simulink model "DconstPQ_snt"  (R2025b)
settings: Solver=ode45  StartTime=0.0  StopTime=10.0  RelTol=1e-3  EnableMultiTasking=on
undefined symbols (not defined in the file or in its folder): DiscIntNeverNeededParam, Ts
libraries: fl_lib x14, nesl_utility x14, mcbeeMathTransformLib x12, eeTransforms x12
(part 1 of 2)
settings Model: Creator=gdudgeon  LastModifiedBy=gdudgeon
settings SolverCC: AlgebraicLoopSolver=TrustRegion
settings DataIOCC: LimitDataPoints=on  SaveFormat=Array  ReturnWorkspaceOutputs=off
settings OptimizationCC: ExpressionDepthLimit=2147483647.0  LifeSpan=inf
settings DebuggingCC: UnderspecifiedInitializationDetection=Classic  MergeDetectMultiDrivingBlocksExec=none  SolverPrmCheckMsg=warning  UnconnectedInputMsg=warning  UnconnectedOutputMsg=warning  UnconnectedLineMsg=warning  StateNameClashWarn=warning  SFUnexpectedBacktrackingDiag=warning  SFNoUnconditionalDefaultTransitionDiag=warning  SFExecutionAtInitializationDiag=none  ArithmeticOperatorsInVariantConditions=warning
settings HardwareCC: ProdBitPerPointer=32.0  ProdBitPerSizeT=32.0  ProdBitPerPtrDiffT=32.0  ProdLargestAtomicFloat=None  ProdIntDivRoundTo=Undefined  ProdEndianess=Unspecified  ProdWordSize=32.0  ProdHWDeviceType=32-bit Generic
settings ModelReferenceCC: EnableRefExpFcnMdlSchedulingChecks=on  PropagateSignalLabelsOutOfModel=off
settings SFSimCC: SimUseLocalCustomCode=off  CustomCodeUndefinedFunction=UseInterfaceOnly
settings RTWCC: RTWUseLocalCustomCode=off  GPUComputeCapability=3.5
settings CodeAppCC: StateflowObjectComments=on
settings GRTTargetCC: TargetLangStandard=C89/C90 (ANSI)
settings ConfigComp: CovMetricSettings=dw  CovSaveCumulativeToWorkspaceVar=on  CovSaveSingleToWorkspaceVar=on  CovExternalEMLEnable=off  CovSFcnEnable=off
settings SimscapeCC: SimscapeNormalizeSystem=off

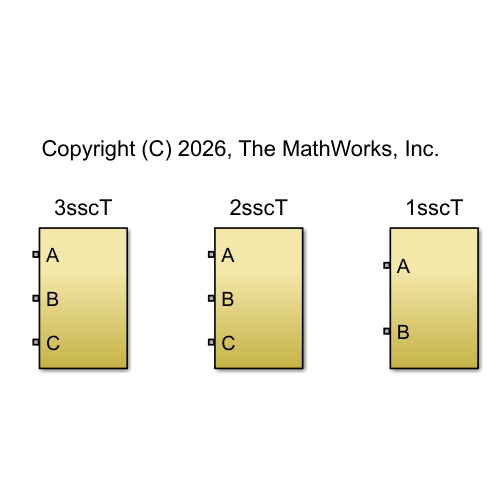
[thumbnail: Simulink's stored preview of the top-level diagram]
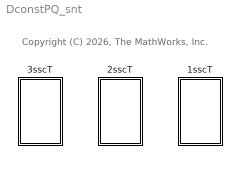
== system DconstPQ_snt ==
  note: Copyright (C) 2026, The MathWorks, Inc.
  1sscT : Subsystem
  2sscT : Subsystem
  3sscT : Subsystem

== system DconstPQ_snt/1sscT ==
  PQ1 : From
  constPQ1 : Subsystem
  A : PMIOPort  Side=Left
  B : PMIOPort  Port=2  Side=Left
  wires:
  PQ1/1 -> constPQ1/1(PQ)
  connections:
  constPQ1/LConn1 -- B/RConn1
  constPQ1/RConn1 -- A/RConn1

== system DconstPQ_snt/2sscT ==
  PQ1 : From
  PQ2 : From
  constPQ : Subsystem  Commented=on
  constPQ1 : Subsystem
  constPQ2 : Subsystem
  A : PMIOPort  Side=Left
  B : PMIOPort  Port=2  Side=Left
  C : PMIOPort  Port=3  Side=Left
  wires:
  PQ2/1 -> constPQ2/1(PQ)
  PQ1/1 -> constPQ1/1(PQ)
  connections:
  constPQ1/RConn1 -- A/RConn1
  B/RConn1 -- constPQ2/RConn1 -- constPQ1/LConn1
  constPQ2/LConn1 -- C/RConn1

== system DconstPQ_snt/3sscT ==
  PQ1 : From
  PQ2 : From
  PQ3 : From
  constPQ1 : Subsystem
  constPQ2 : Subsystem
  constPQ3 : Subsystem
  A : PMIOPort  Side=Left
  B : PMIOPort  Port=2  Side=Left
  C : PMIOPort  Port=3  Side=Left
  wires:
  PQ3/1 -> constPQ3/1(PQ)
  PQ2/1 -> constPQ2/1(PQ)
  PQ1/1 -> constPQ1/1(PQ)
  connections:
  C/RConn1 -- constPQ3/RConn1 -- constPQ2/LConn1
  B/RConn1 -- constPQ2/RConn1 -- constPQ1/LConn1
  A/RConn1 -- constPQ3/LConn1 -- constPQ1/RConn1

== system DconstPQ_snt/1sscT/constPQ1 ==
  PQ : Inport
  Controlled Current Source : fl_lib/Electrical/Electrical Sources/Controlled Current Source
  Demux : Demux  Outputs=2
  PS-Simulink Converter : nesl_utility/PS-Simulink Converter  PhysicalDomain=network_engine_domain  SubClassName=ps_output  LeftPortType=input  RightPortType=output  PseudoPeriodic=off  Frequencies=[]  VectorFormat=inherit  Unit=inherit  AffineConversion=off
  Simulink-PS Converter : nesl_utility/Simulink-PS Converter  PhysicalDomain=network_engine_domain  SubClassName=ps_input  LeftPortType=input  RightPortType=output  PseudoPeriodic=off  Frequencies=[]  NoiseDistribution=none  NoiseParameters=[]  Unit=1  AffineConversion=off  FilteringAndDerivatives=zero  SimscapeFilterOrder=1  InputFilterTimeConstant=0.001  UdotUserProvided=0
  Voltage Sensor : fl_lib/Electrical/Electrical Sensors/Voltage Sensor
  single-phase PQ : Subsystem
      settings: PortSchema="{\"entries\":[{\"content\":{\"sides\":[{\"content\":{\"connectorIds\":[\"In1\",\"In2\"]},\"type\":\"ConnectorPlacement.EquallySpacedRectSide\",\"uuid\":\"dcb77ad6-d65a-4afe-9b75-44cea2e03bc8\"},{\"content\":{\"connectorIds\":[\"Out1\"],\"side\":\"RIGHT\"},\"type\":\"ConnectorPlacement.EquallySpacedRectSide\",\"uuid\":\"20550ec8-912f-4e6b-8efc-55d7f6680ac4\"},{\"content\":{\"side\":\"TOP\"},\"type\":\"ConnectorPlacement.EquallySpacedRectSide\",\"uuid\":\"6ad8cbf4-1495-4620-97d9-4b8af34d00d1\"},{\"content\":{\"connectorIds\":[\"In3\"],\"side\":\"BOTTOM\"},\"type\":\"ConnectorPlacement.EquallySpacedRectSide\",\"uuid\":\"0b9a8788-8400-4a69-9d07-dd0028530e33\"}]},\"type\":\"ConnectorPlacement.EquallySpacedConnector\",\"uuid\":\"b57ec49b-aa32-43b3-a026-14ed90072d63\"}],\"packageUris\":[\"http://schema.mathworks.com/mf0/Connector/R2020b\"],\"version\":\"1.0\"}"
  + : PMIOPort  Side=Right
  - : PMIOPort  Port=2  Side=Left
  wires:
  PS-Simulink Converter/1 -> single-phase PQ/3(meas)
  single-phase PQ/1(I_1ph) -> Simulink-PS Converter/1
  Demux/1 -> single-phase PQ/1(P)
  Demux/2 -> single-phase PQ/2(Q)
  PQ/1 -> Demux/1
  connections:
  Controlled Current Source/RConn2 -- -/RConn1 -- Voltage Sensor/RConn2
  Voltage Sensor/LConn1 -- +/RConn1 -- Controlled Current Source/LConn1
  PS-Simulink Converter/LConn1 -- Voltage Sensor/RConn1
  Simulink-PS Converter/RConn1 -- Controlled Current Source/RConn1

== system DconstPQ_snt/2sscT/constPQ ==
  PQ : Inport
  Controlled Current Source : fl_lib/Electrical/Electrical Sources/Controlled Current Source
  Demux : Demux  Outputs=2
  PS-Simulink Converter : nesl_utility/PS-Simulink Converter  PhysicalDomain=network_engine_domain  SubClassName=ps_output  LeftPortType=input  RightPortType=output  PseudoPeriodic=off  Frequencies=[]  VectorFormat=inherit  Unit=inherit  AffineConversion=off
  Simulink-PS Converter : nesl_utility/Simulink-PS Converter  PhysicalDomain=network_engine_domain  SubClassName=ps_input  LeftPortType=input  RightPortType=output  PseudoPeriodic=off  Frequencies=[]  NoiseDistribution=none  NoiseParameters=[]  Unit=1  AffineConversion=off  FilteringAndDerivatives=zero  SimscapeFilterOrder=1  InputFilterTimeConstant=0.001  UdotUserProvided=0
  Voltage Sensor : fl_lib/Electrical/Electrical Sensors/Voltage Sensor
  single-phase PQ : Subsystem
      settings: PortSchema="{\"entries\":[{\"content\":{\"sides\":[{\"content\":{\"connectorIds\":[\"In1\",\"In2\"]},\"type\":\"ConnectorPlacement.EquallySpacedRectSide\",\"uuid\":\"dcb77ad6-d65a-4afe-9b75-44cea2e03bc8\"},{\"content\":{\"connectorIds\":[\"Out1\"],\"side\":\"RIGHT\"},\"type\":\"ConnectorPlacement.EquallySpacedRectSide\",\"uuid\":\"20550ec8-912f-4e6b-8efc-55d7f6680ac4\"},{\"content\":{\"side\":\"TOP\"},\"type\":\"ConnectorPlacement.EquallySpacedRectSide\",\"uuid\":\"6ad8cbf4-1495-4620-97d9-4b8af34d00d1\"},{\"content\":{\"connectorIds\":[\"In3\"],\"side\":\"BOTTOM\"},\"type\":\"ConnectorPlacement.EquallySpacedRectSide\",\"uuid\":\"0b9a8788-8400-4a69-9d07-dd0028530e33\"}]},\"type\":\"ConnectorPlacement.EquallySpacedConnector\",\"uuid\":\"b57ec49b-aa32-43b3-a026-14ed90072d63\"}],\"packageUris\":[\"http://schema.mathworks.com/mf0/Connector/R2020b\"],\"version\":\"1.0\"}"
  + : PMIOPort  Side=Right
  - : PMIOPort  Port=2  Side=Left
  wires:
  PS-Simulink Converter/1 -> single-phase PQ/3(meas)
  single-phase PQ/1(I_1ph) -> Simulink-PS Converter/1
  Demux/1 -> single-phase PQ/1(P)
  Demux/2 -> single-phase PQ/2(Q)
  PQ/1 -> Demux/1
  connections:
  Controlled Current Source/RConn2 -- -/RConn1 -- Voltage Sensor/RConn2
  Voltage Sensor/LConn1 -- +/RConn1 -- Controlled Current Source/LConn1
  PS-Simulink Converter/LConn1 -- Voltage Sensor/RConn1
  Simulink-PS Converter/RConn1 -- Controlled Current Source/RConn1

== system DconstPQ_snt/2sscT/constPQ1 ==
  PQ : Inport
  Controlled Current Source : fl_lib/Electrical/Electrical Sources/Controlled Current Source
  Demux : Demux  Outputs=2
  PS-Simulink Converter : nesl_utility/PS-Simulink Converter  PhysicalDomain=network_engine_domain  SubClassName=ps_output  LeftPortType=input  RightPortType=output  PseudoPeriodic=off  Frequencies=[]  VectorFormat=inherit  Unit=inherit  AffineConversion=off
  Simulink-PS Converter : nesl_utility/Simulink-PS Converter  PhysicalDomain=network_engine_domain  SubClassName=ps_input  LeftPortType=input  RightPortType=output  PseudoPeriodic=off  Frequencies=[]  NoiseDistribution=none  NoiseParameters=[]  Unit=1  AffineConversion=off  FilteringAndDerivatives=zero  SimscapeFilterOrder=1  InputFilterTimeConstant=0.001  UdotUserProvided=0
  Voltage Sensor : fl_lib/Electrical/Electrical Sensors/Voltage Sensor
  single-phase PQ : Subsystem
      settings: PortSchema="{\"entries\":[{\"content\":{\"sides\":[{\"content\":{\"connectorIds\":[\"In1\",\"In2\"]},\"type\":\"ConnectorPlacement.EquallySpacedRectSide\",\"uuid\":\"dcb77ad6-d65a-4afe-9b75-44cea2e03bc8\"},{\"content\":{\"connectorIds\":[\"Out1\"],\"side\":\"RIGHT\"},\"type\":\"ConnectorPlacement.EquallySpacedRectSide\",\"uuid\":\"20550ec8-912f-4e6b-8efc-55d7f6680ac4\"},{\"content\":{\"side\":\"TOP\"},\"type\":\"ConnectorPlacement.EquallySpacedRectSide\",\"uuid\":\"6ad8cbf4-1495-4620-97d9-4b8af34d00d1\"},{\"content\":{\"connectorIds\":[\"In3\"],\"side\":\"BOTTOM\"},\"type\":\"ConnectorPlacement.EquallySpacedRectSide\",\"uuid\":\"0b9a8788-8400-4a69-9d07-dd0028530e33\"}]},\"type\":\"ConnectorPlacement.EquallySpacedConnector\",\"uuid\":\"b57ec49b-aa32-43b3-a026-14ed90072d63\"}],\"packageUris\":[\"http://schema.mathworks.com/mf0/Connector/R2020b\"],\"version\":\"1.0\"}"
  + : PMIOPort  Side=Right
  - : PMIOPort  Port=2  Side=Left
  wires:
  PS-Simulink Converter/1 -> single-phase PQ/3(meas)
  single-phase PQ/1(I_1ph) -> Simulink-PS Converter/1
  Demux/1 -> single-phase PQ/1(P)
  Demux/2 -> single-phase PQ/2(Q)
  PQ/1 -> Demux/1
  connections:
  Controlled Current Source/RConn2 -- -/RConn1 -- Voltage Sensor/RConn2
  Voltage Sensor/LConn1 -- +/RConn1 -- Controlled Current Source/LConn1
  PS-Simulink Converter/LConn1 -- Voltage Sensor/RConn1
  Simulink-PS Converter/RConn1 -- Controlled Current Source/RConn1

== system DconstPQ_snt/2sscT/constPQ2 ==
  PQ : Inport
  Controlled Current Source : fl_lib/Electrical/Electrical Sources/Controlled Current Source
  Demux : Demux  Outputs=2
  PS-Simulink Converter : nesl_utility/PS-Simulink Converter  PhysicalDomain=network_engine_domain  SubClassName=ps_output  LeftPortType=input  RightPortType=output  PseudoPeriodic=off  Frequencies=[]  VectorFormat=inherit  Unit=inherit  AffineConversion=off
  Simulink-PS Converter : nesl_utility/Simulink-PS Converter  PhysicalDomain=network_engine_domain  SubClassName=ps_input  LeftPortType=input  RightPortType=output  PseudoPeriodic=off  Frequencies=[]  NoiseDistribution=none  NoiseParameters=[]  Unit=1  AffineConversion=off  FilteringAndDerivatives=zero  SimscapeFilterOrder=1  InputFilterTimeConstant=0.001  UdotUserProvided=0
  Voltage Sensor : fl_lib/Electrical/Electrical Sensors/Voltage Sensor
  single-phase PQ : Subsystem
      settings: PortSchema="{\"entries\":[{\"content\":{\"sides\":[{\"content\":{\"connectorIds\":[\"In1\",\"In2\"]},\"type\":\"ConnectorPlacement.EquallySpacedRectSide\",\"uuid\":\"dcb77ad6-d65a-4afe-9b75-44cea2e03bc8\"},{\"content\":{\"connectorIds\":[\"Out1\"],\"side\":\"RIGHT\"},\"type\":\"ConnectorPlacement.EquallySpacedRectSide\",\"uuid\":\"20550ec8-912f-4e6b-8efc-55d7f6680ac4\"},{\"content\":{\"side\":\"TOP\"},\"type\":\"ConnectorPlacement.EquallySpacedRectSide\",\"uuid\":\"6ad8cbf4-1495-4620-97d9-4b8af34d00d1\"},{\"content\":{\"connectorIds\":[\"In3\"],\"side\":\"BOTTOM\"},\"type\":\"ConnectorPlacement.EquallySpacedRectSide\",\"uuid\":\"0b9a8788-8400-4a69-9d07-dd0028530e33\"}]},\"type\":\"ConnectorPlacement.EquallySpacedConnector\",\"uuid\":\"b57ec49b-aa32-43b3-a026-14ed90072d63\"}],\"packageUris\":[\"http://schema.mathworks.com/mf0/Connector/R2020b\"],\"version\":\"1.0\"}"
  + : PMIOPort  Side=Right
  - : PMIOPort  Port=2  Side=Left
  wires:
  PQ/1 -> Demux/1
  Demux/2 -> single-phase PQ/2(Q)
  Demux/1 -> single-phase PQ/1(P)
  single-phase PQ/1(I_1ph) -> Simulink-PS Converter/1
  PS-Simulink Converter/1 -> single-phase PQ/3(meas)
  connections:
  Simulink-PS Converter/RConn1 -- Controlled Current Source/RConn1
  PS-Simulink Converter/LConn1 -- Voltage Sensor/RConn1
  Controlled Current Source/LConn1 -- +/RConn1 -- Voltage Sensor/LConn1
  Voltage Sensor/RConn2 -- -/RConn1 -- Controlled Current Source/RConn2

== system DconstPQ_snt/3sscT/constPQ1 ==
  PQ : Inport
  Controlled Current Source : fl_lib/Electrical/Electrical Sources/Controlled Current Source
  Demux : Demux  Outputs=2
  PS-Simulink Converter : nesl_utility/PS-Simulink Converter  PhysicalDomain=network_engine_domain  SubClassName=ps_output  LeftPortType=input  RightPortType=output  PseudoPeriodic=off  Frequencies=[]  VectorFormat=inherit  Unit=inherit  AffineConversion=off
  Simulink-PS Converter : nesl_utility/Simulink-PS Converter  PhysicalDomain=network_engine_domain  SubClassName=ps_input  LeftPortType=input  RightPortType=output  PseudoPeriodic=off  Frequencies=[]  NoiseDistribution=none  NoiseParameters=[]  Unit=1  AffineConversion=off  FilteringAndDerivatives=zero  SimscapeFilterOrder=1  InputFilterTimeConstant=0.001  UdotUserProvided=0
  Voltage Sensor : fl_lib/Electrical/Electrical Sensors/Voltage Sensor
  single-phase PQ : Subsystem
      settings: PortSchema="{\"entries\":[{\"content\":{\"sides\":[{\"content\":{\"connectorIds\":[\"In1\",\"In2\"]},\"type\":\"ConnectorPlacement.EquallySpacedRectSide\",\"uuid\":\"dcb77ad6-d65a-4afe-9b75-44cea2e03bc8\"},{\"content\":{\"connectorIds\":[\"Out1\"],\"side\":\"RIGHT\"},\"type\":\"ConnectorPlacement.EquallySpacedRectSide\",\"uuid\":\"20550ec8-912f-4e6b-8efc-55d7f6680ac4\"},{\"content\":{\"side\":\"TOP\"},\"type\":\"ConnectorPlacement.EquallySpacedRectSide\",\"uuid\":\"6ad8cbf4-1495-4620-97d9-4b8af34d00d1\"},{\"content\":{\"connectorIds\":[\"In3\"],\"side\":\"BOTTOM\"},\"type\":\"ConnectorPlacement.EquallySpacedRectSide\",\"uuid\":\"0b9a8788-8400-4a69-9d07-dd0028530e33\"}]},\"type\":\"ConnectorPlacement.EquallySpacedConnector\",\"uuid\":\"b57ec49b-aa32-43b3-a026-14ed90072d63\"}],\"packageUris\":[\"http://schema.mathworks.com/mf0/Connector/R2020b\"],\"version\":\"1.0\"}"
  + : PMIOPort  Side=Right
  - : PMIOPort  Port=2  Side=Left
  wires:
  PS-Simulink Converter/1 -> single-phase PQ/3(meas)
  single-phase PQ/1(I_1ph) -> Simulink-PS Converter/1
  Demux/1 -> single-phase PQ/1(P)
  Demux/2 -> single-phase PQ/2(Q)
  PQ/1 -> Demux/1
  connections:
  Controlled Current Source/RConn2 -- -/RConn1 -- Voltage Sensor/RConn2
  Voltage Sensor/LConn1 -- +/RConn1 -- Controlled Current Source/LConn1
  PS-Simulink Converter/LConn1 -- Voltage Sensor/RConn1
  Simulink-PS Converter/RConn1 -- Controlled Current Source/RConn1

== system DconstPQ_snt/3sscT/constPQ2 ==
  PQ : Inport
  Controlled Current Source : fl_lib/Electrical/Electrical Sources/Controlled Current Source
  Demux : Demux  Outputs=2
  PS-Simulink Converter : nesl_utility/PS-Simulink Converter  PhysicalDomain=network_engine_domain  SubClassName=ps_output  LeftPortType=input  RightPortType=output  PseudoPeriodic=off  Frequencies=[]  VectorFormat=inherit  Unit=inherit  AffineConversion=off
  Simulink-PS Converter : nesl_utility/Simulink-PS Converter  PhysicalDomain=network_engine_domain  SubClassName=ps_input  LeftPortType=input  RightPortType=output  PseudoPeriodic=off  Frequencies=[]  NoiseDistribution=none  NoiseParameters=[]  Unit=1  AffineConversion=off  FilteringAndDerivatives=zero  SimscapeFilterOrder=1  InputFilterTimeConstant=0.001  UdotUserProvided=0
  Voltage Sensor : fl_lib/Electrical/Electrical Sensors/Voltage Sensor
  single-phase PQ : Subsystem
      settings: PortSchema="{\"entries\":[{\"content\":{\"sides\":[{\"content\":{\"connectorIds\":[\"In1\",\"In2\"]},\"type\":\"ConnectorPlacement.EquallySpacedRectSide\",\"uuid\":\"dcb77ad6-d65a-4afe-9b75-44cea2e03bc8\"},{\"content\":{\"connectorIds\":[\"Out1\"],\"side\":\"RIGHT\"},\"type\":\"ConnectorPlacement.EquallySpacedRectSide\",\"uuid\":\"20550ec8-912f-4e6b-8efc-55d7f6680ac4\"},{\"content\":{\"side\":\"TOP\"},\"type\":\"ConnectorPlacement.EquallySpacedRectSide\",\"uuid\":\"6ad8cbf4-1495-4620-97d9-4b8af34d00d1\"},{\"content\":{\"connectorIds\":[\"In3\"],\"side\":\"BOTTOM\"},\"type\":\"ConnectorPlacement.EquallySpacedRectSide\",\"uuid\":\"0b9a8788-8400-4a69-9d07-dd0028530e33\"}]},\"type\":\"ConnectorPlacement.EquallySpacedConnector\",\"uuid\":\"b57ec49b-aa32-43b3-a026-14ed90072d63\"}],\"packageUris\":[\"http://schema.mathworks.com/mf0/Connector/R2020b\"],\"version\":\"1.0\"}"
  + : PMIOPort  Side=Right
  - : PMIOPort  Port=2  Side=Left
  wires:
  PQ/1 -> Demux/1
  Demux/2 -> single-phase PQ/2(Q)
  Demux/1 -> single-phase PQ/1(P)
  single-phase PQ/1(I_1ph) -> Simulink-PS Converter/1
  PS-Simulink Converter/1 -> single-phase PQ/3(meas)
  connections:
  Simulink-PS Converter/RConn1 -- Controlled Current Source/RConn1
  PS-Simulink Converter/LConn1 -- Voltage Sensor/RConn1
  Controlled Current Source/LConn1 -- +/RConn1 -- Voltage Sensor/LConn1
  Voltage Sensor/RConn2 -- -/RConn1 -- Controlled Current Source/RConn2

== system DconstPQ_snt/3sscT/constPQ3 ==
  PQ : Inport
  Controlled Current Source : fl_lib/Electrical/Electrical Sources/Controlled Current Source
  Demux : Demux  Outputs=2
  PS-Simulink Converter : nesl_utility/PS-Simulink Converter  PhysicalDomain=network_engine_domain  SubClassName=ps_output  LeftPortType=input  RightPortType=output  PseudoPeriodic=off  Frequencies=[]  VectorFormat=inherit  Unit=inherit  AffineConversion=off
  Simulink-PS Converter : nesl_utility/Simulink-PS Converter  PhysicalDomain=network_engine_domain  SubClassName=ps_input  LeftPortType=input  RightPortType=output  PseudoPeriodic=off  Frequencies=[]  NoiseDistribution=none  NoiseParameters=[]  Unit=1  AffineConversion=off  FilteringAndDerivatives=zero  SimscapeFilterOrder=1  InputFilterTimeConstant=0.001  UdotUserProvided=0
  Voltage Sensor : fl_lib/Electrical/Electrical Sensors/Voltage Sensor
  single-phase PQ : Subsystem
      settings: PortSchema="{\"entries\":[{\"content\":{\"sides\":[{\"content\":{\"connectorIds\":[\"In1\",\"In2\"]},\"type\":\"ConnectorPlacement.EquallySpacedRectSide\",\"uuid\":\"dcb77ad6-d65a-4afe-9b75-44cea2e03bc8\"},{\"content\":{\"connectorIds\":[\"Out1\"],\"side\":\"RIGHT\"},\"type\":\"ConnectorPlacement.EquallySpacedRectSide\",\"uuid\":\"20550ec8-912f-4e6b-8efc-55d7f6680ac4\"},{\"content\":{\"side\":\"TOP\"},\"type\":\"ConnectorPlacement.EquallySpacedRectSide\",\"uuid\":\"6ad8cbf4-1495-4620-97d9-4b8af34d00d1\"},{\"content\":{\"connectorIds\":[\"In3\"],\"side\":\"BOTTOM\"},\"type\":\"ConnectorPlacement.EquallySpacedRectSide\",\"uuid\":\"0b9a8788-8400-4a69-9d07-dd0028530e33\"}]},\"type\":\"ConnectorPlacement.EquallySpacedConnector\",\"uuid\":\"b57ec49b-aa32-43b3-a026-14ed90072d63\"}],\"packageUris\":[\"http://schema.mathworks.com/mf0/Connector/R2020b\"],\"version\":\"1.0\"}"
  + : PMIOPort  Side=Right
  - : PMIOPort  Port=2  Side=Left
  wires:
  PS-Simulink Converter/1 -> single-phase PQ/3(meas)
  single-phase PQ/1(I_1ph) -> Simulink-PS Converter/1
  Demux/1 -> single-phase PQ/1(P)
  Demux/2 -> single-phase PQ/2(Q)
  PQ/1 -> Demux/1
  connections:
  Controlled Current Source/RConn2 -- -/RConn1 -- Voltage Sensor/RConn2
  Voltage Sensor/LConn1 -- +/RConn1 -- Controlled Current Source/LConn1
  PS-Simulink Converter/LConn1 -- Voltage Sensor/RConn1
  Simulink-PS Converter/RConn1 -- Controlled Current Source/RConn1

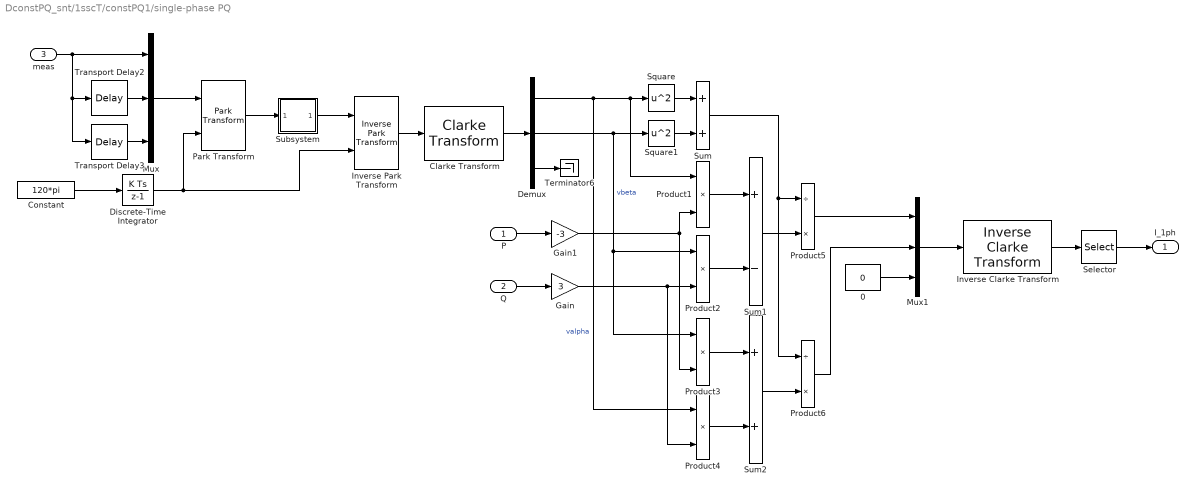
== system DconstPQ_snt/1sscT/constPQ1/single-phase PQ ==
  P : Inport
  Q : Inport  Port=2
  meas : Inport  Port=3
  "0 " : Constant  Value=0  VectorParams1D=off  SampleTime=Ts
  Clarke Transform : mcbeeMathTransformLib/Clarke Transform  PowerInvariant=on  UseWithEmbedded=off  PhaseInput=Two inputs
      settings: LibrarySourceBlock=|
      | ee_sl_lib/Mathematical
      | Transforms/Clarke Transform
  Constant : Constant  Value=120*pi  VectorParams1D=off  SampleTime=Ts
  Demux : Demux  Outputs=3
  Discrete-Time Integrator : DiscreteIntegrator  SampleTime=Ts  ICPrevOutput=DiscIntNeverNeededParam  ICPrevScaledInput=DiscIntNeverNeededParam
  Gain : Gain  Gain=3
  Gain1 : Gain  Gain=-3
  Inverse Clarke Transform : mcbeeMathTransformLib/Inverse Clarke Transform  PowerInvariant=on  UseWithEmbedded=off  PhaseInput=Two inputs
      settings: LibrarySourceBlock=|
      | ee_sl_lib/Mathematical
      | Transforms/Inverse
      | Clarke Transform
  Inverse Park Transform : eeTransforms/Inverse Park Transform  AxisAlignment=Q-axis  PowerInvariant=off
      settings: LibrarySourceBlock=|
      | ee_sl_lib/Mathematical
      | Transforms/Inverse
      | Park Transform
  Mux : Mux  Inputs=3
  Mux1 : Mux  Inputs=3
  Park Transform : eeTransforms/Park Transform  AxisAlignment=Q-axis  PowerInvariant=off
      settings: LibrarySourceBlock=|
      | ee_sl_lib/Mathematical
      | Transforms/Park Transform
  Product{1..4} (4 alike) : Product
  Product5 : Product  Inputs=/*
  Product6 : Product  Inputs=/*
  Selector : Selector  InputPortWidth=3  IndexOptions=Index vector (dialog)  Indices=1  OutputSizes=1
  Square : Math  Operator=square
  Square1 : Math  Operator=square
  Subsystem : Subsystem
  Sum : Sum
  Sum1 : Sum  Inputs=+-
  Sum2 : Sum
  Terminator6 : Terminator
  Transport Delay2 : TransportDelay  DelayTime=1/180
  Transport Delay3 : TransportDelay  DelayTime=2/180
  I_1ph : Outport
  wires:
  Sum2/1 -> Product6/2
  Sum/1 -> Product5/1, Product6/1
  P/1 -> Gain1/1
  Square1/1 -> Sum/2
  Product3/1 -> Sum2/1
  Demux/2 -> Product3/1, Product2/1, Square1/1  "vbeta"
  Q/1 -> Gain/1
  "0 "/1 -> Mux1/3
  Sum1/1 -> Product5/2
  Product2/1 -> Sum1/2
  Demux/1 -> Product4/1, Product1/1, Square/1  "valpha"
  Product6/1 -> Mux1/2
  Product4/1 -> Sum2/2
  Product1/1 -> Sum1/1
  Square/1 -> Sum/1
  Product5/1 -> Mux1/1
  Constant/1 -> Discrete-Time Integrator/1
  Discrete-Time Integrator/1 -> Park Transform/2, Inverse Park Transform/2
  Subsystem/1(Out1) -> Inverse Park Transform/1
  Transport Delay3/1 -> Mux/3
  meas/1 -> Transport Delay3/1, Transport Delay2/1, Mux/1
  Transport Delay2/1 -> Mux/2
  Gain/1 -> Product4/2, Product2/2
  Gain1/1 -> Product1/2, Product3/2
  Mux/1 -> Park Transform/1
  Selector/1 -> I_1ph/1
  Park Transform/1 -> Subsystem/1(In1)
  Inverse Park Transform/1 -> Clarke Transform/1
  Clarke Transform/1 -> Demux/1
  Demux/3 -> Terminator6/1
  Mux1/1 -> Inverse Clarke Transform/1
  Inverse Clarke Transform/1 -> Selector/1

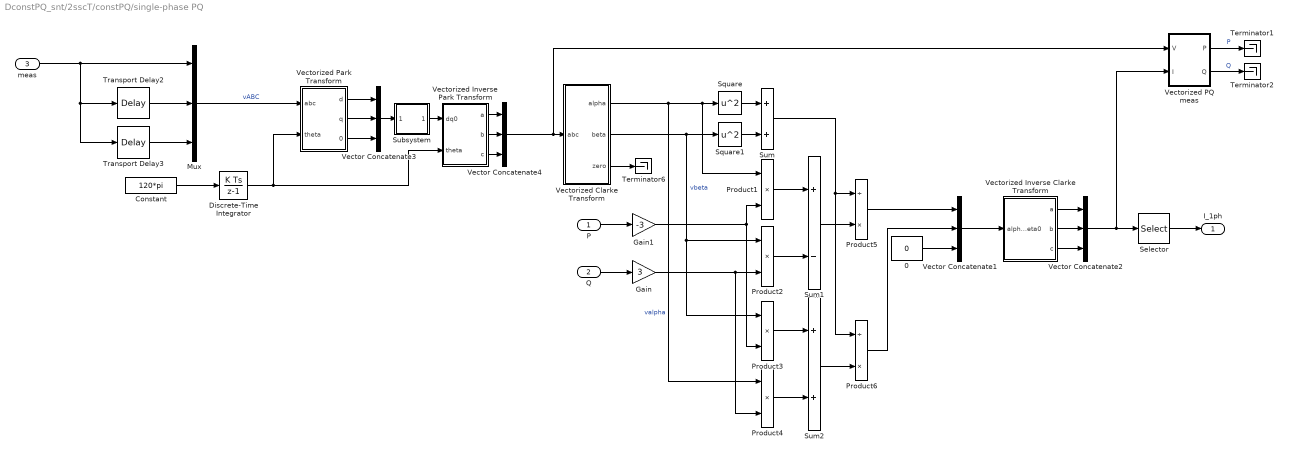
== system DconstPQ_snt/2sscT/constPQ/single-phase PQ ==
  P : Inport
  Q : Inport  Port=2
  meas : Inport  Port=3
  "0 " : Constant  Value=0  VectorParams1D=off  SampleTime=Ts
  Constant : Constant  Value=120*pi  VectorParams1D=off  SampleTime=Ts
  Discrete-Time Integrator : DiscreteIntegrator  SampleTime=Ts  ICPrevOutput=DiscIntNeverNeededParam  ICPrevScaledInput=DiscIntNeverNeededParam
  Gain : Gain  Gain=3
  Gain1 : Gain  Gain=-3
  Mux : Mux  Inputs=3
  Product{1..4} (4 alike) : Product
  Product5 : Product  Inputs=/*
  Product6 : Product  Inputs=/*
  Selector : Selector  InputPortWidth=3  IndexOptions=Index vector (dialog)  Indices=1  OutputSizes=1
  Square : Math  Operator=square
  Square1 : Math  Operator=square
  Subsystem : Subsystem
  Sum : Sum
  Sum1 : Sum  Inputs=+-
  Sum2 : Sum
  Terminator1 : Terminator
  Terminator2 : Terminator
  Terminator6 : Terminator
  Transport Delay2 : TransportDelay  DelayTime=1/180
  Transport Delay3 : TransportDelay  DelayTime=2/180
  Vector Concatenate{1..4} (4 alike) : Concatenate  NumInputs=3  Mode=Multidimensional array
  Vectorized Clarke Transform : Subsystem  mask{no_meas=1}
      mask prompts: no_meas "Number of measurements"
  Vectorized PQ meas : Subsystem  DialogController=POWERSYS.PowerSysDialog
  Vectorized Park Transform : Subsystem  mask{no_meas=1}
      mask prompts: no_meas "Number of measurements"
  Vectorized Inverse Clarke Transform : Subsystem  mask{no_meas=1}
      mask prompts: no_meas "Number of Measurements"
      mask Display:
      | port_label('input', 1, '\alpha\beta0', 'texmode', 'on')
      | port_label('output',1,'a')
      | port_label('output',2,'b')
      | port_label('output',3,'c')
  Vectorized Inverse Park Transform : Subsystem  mask{no_meas=1}
      mask prompts: no_meas "Number of Measurements"
  I_1ph : Outport
  wires:
  Sum2/1 -> Product6/2
  Sum/1 -> Product5/1, Product6/1
  P/1 -> Gain1/1
  Square1/1 -> Sum/2
  Product3/1 -> Sum2/1
  Vectorized Clarke Transform/2(beta) -> Product3/1, Product2/1, Square1/1  "vbeta"
  Q/1 -> Gain/1
  "0 "/1 -> Vector Concatenate1/3
  Sum1/1 -> Product5/2
  Vectorized Inverse Clarke Transform/1(a) -> Vector Concatenate2/1
  Vectorized Inverse Clarke Transform/2(b) -> Vector Concatenate2/2
  Vectorized Clarke Transform/3(zero) -> Terminator6/1
  Product2/1 -> Sum1/2
  Vectorized Clarke Transform/1(alpha) -> Product4/1, Product1/1, Square/1  "valpha"
  Product6/1 -> Vector Concatenate1/2
  Product4/1 -> Sum2/2
  Vectorized Inverse Clarke Transform/3(c) -> Vector Concatenate2/3
  Product1/1 -> Sum1/1
  Vector Concatenate1/1 -> Vectorized Inverse Clarke Transform/1(alphabeta0)
  Square/1 -> Sum/1
  Product5/1 -> Vector Concatenate1/1
  Vectorized PQ meas/1(P) -> Terminator1/1  "P"
  Vectorized PQ meas/2(Q) -> Terminator2/1  "Q"
  Vector Concatenate2/1 -> Selector/1, Vectorized PQ meas/2(I)
  Vectorized Park Transform/1(d) -> Vector Concatenate3/1
  Vectorized Park Transform/2(q) -> Vector Concatenate3/2
  Vectorized Park Transform/3(0) -> Vector Concatenate3/3
  Vectorized Inverse Park Transform/1(a) -> Vector Concatenate4/1
  Vectorized Inverse Park Transform/2(b) -> Vector Concatenate4/2
  Vectorized Inverse Park Transform/3(c) -> Vector Concatenate4/3
  Vector Concatenate4/1 -> Vectorized Clarke Transform/1(abc), Vectorized PQ meas/1(V)
  Constant/1 -> Discrete-Time Integrator/1
  Discrete-Time Integrator/1 -> Vectorized Inverse Park Transform/2(theta), Vectorized Park Transform/2(theta)
  Vector Concatenate3/1 -> Subsystem/1(In1)
  Subsystem/1(Out1) -> Vectorized Inverse Park Transform/1(dq0)
  Transport Delay3/1 -> Mux/3
  meas/1 -> Transport Delay3/1, Transport Delay2/1, Mux/1
  Transport Delay2/1 -> Mux/2
  Gain/1 -> Product4/2, Product2/2
  Gain1/1 -> Product1/2, Product3/2
  Mux/1 -> Vectorized Park Transform/1(abc)  "vABC"
  Selector/1 -> I_1ph/1

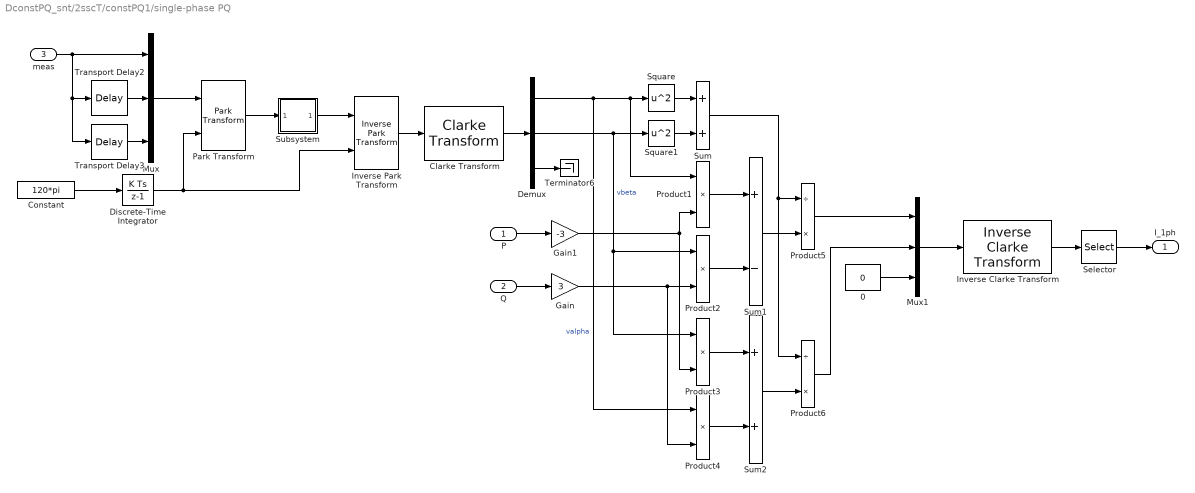
== system DconstPQ_snt/2sscT/constPQ1/single-phase PQ ==
  P : Inport
  Q : Inport  Port=2
  meas : Inport  Port=3
  "0 " : Constant  Value=0  VectorParams1D=off  SampleTime=Ts
  Clarke Transform : mcbeeMathTransformLib/Clarke Transform  PowerInvariant=on  UseWithEmbedded=off  PhaseInput=Two inputs
      settings: LibrarySourceBlock=|
      | ee_sl_lib/Mathematical
      | Transforms/Clarke Transform
  Constant : Constant  Value=120*pi  VectorParams1D=off  SampleTime=Ts
  Demux : Demux  Outputs=3
  Discrete-Time Integrator : DiscreteIntegrator  SampleTime=Ts  ICPrevOutput=DiscIntNeverNeededParam  ICPrevScaledInput=DiscIntNeverNeededParam
  Gain : Gain  Gain=3
  Gain1 : Gain  Gain=-3
  Inverse Clarke Transform : mcbeeMathTransformLib/Inverse Clarke Transform  PowerInvariant=on  UseWithEmbedded=off  PhaseInput=Two inputs
      settings: LibrarySourceBlock=|
      | ee_sl_lib/Mathematical
      | Transforms/Inverse
      | Clarke Transform
  Inverse Park Transform : eeTransforms/Inverse Park Transform  AxisAlignment=Q-axis  PowerInvariant=off
      settings: LibrarySourceBlock=|
      | ee_sl_lib/Mathematical
      | Transforms/Inverse
      | Park Transform
  Mux : Mux  Inputs=3
  Mux1 : Mux  Inputs=3
  Park Transform : eeTransforms/Park Transform  AxisAlignment=Q-axis  PowerInvariant=off
      settings: LibrarySourceBlock=|
      | ee_sl_lib/Mathematical
      | Transforms/Park Transform
  Product{1..4} (4 alike) : Product
  Product5 : Product  Inputs=/*
  Product6 : Product  Inputs=/*
  Selector : Selector  InputPortWidth=3  IndexOptions=Index vector (dialog)  Indices=1  OutputSizes=1
  Square : Math  Operator=square
  Square1 : Math  Operator=square
  Subsystem : Subsystem
  Sum : Sum
  Sum1 : Sum  Inputs=+-
  Sum2 : Sum
  Terminator6 : Terminator
  Transport Delay2 : TransportDelay  DelayTime=1/180
  Transport Delay3 : TransportDelay  DelayTime=2/180
  I_1ph : Outport
  wires:
  Sum2/1 -> Product6/2
  Sum/1 -> Product5/1, Product6/1
  P/1 -> Gain1/1
  Square1/1 -> Sum/2
  Product3/1 -> Sum2/1
  Demux/2 -> Product3/1, Product2/1, Square1/1  "vbeta"
  Q/1 -> Gain/1
  "0 "/1 -> Mux1/3
  Sum1/1 -> Product5/2
  Product2/1 -> Sum1/2
  Demux/1 -> Product4/1, Product1/1, Square/1  "valpha"
  Product6/1 -> Mux1/2
  Product4/1 -> Sum2/2
  Product1/1 -> Sum1/1
  Square/1 -> Sum/1
  Product5/1 -> Mux1/1
  Constant/1 -> Discrete-Time Integrator/1
  Discrete-Time Integrator/1 -> Park Transform/2, Inverse Park Transform/2
  Subsystem/1(Out1) -> Inverse Park Transform/1
  Transport Delay3/1 -> Mux/3
  meas/1 -> Transport Delay3/1, Transport Delay2/1, Mux/1
  Transport Delay2/1 -> Mux/2
  Gain/1 -> Product4/2, Product2/2
  Gain1/1 -> Product1/2, Product3/2
  Mux/1 -> Park Transform/1
  Selector/1 -> I_1ph/1
  Park Transform/1 -> Subsystem/1(In1)
  Inverse Park Transform/1 -> Clarke Transform/1
  Clarke Transform/1 -> Demux/1
  Demux/3 -> Terminator6/1
  Mux1/1 -> Inverse Clarke Transform/1
  Inverse Clarke Transform/1 -> Selector/1

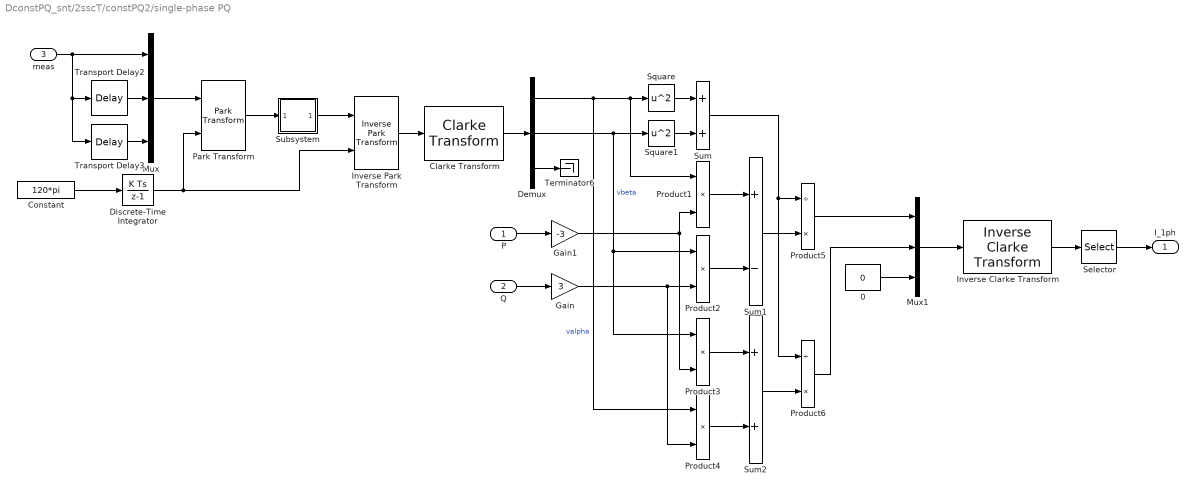
== system DconstPQ_snt/2sscT/constPQ2/single-phase PQ ==
  P : Inport
  Q : Inport  Port=2
  meas : Inport  Port=3
  "0 " : Constant  Value=0  VectorParams1D=off  SampleTime=Ts
  Clarke Transform : mcbeeMathTransformLib/Clarke Transform  PowerInvariant=on  UseWithEmbedded=off  PhaseInput=Two inputs
      settings: LibrarySourceBlock=|
      | ee_sl_lib/Mathematical
      | Transforms/Clarke Transform
  Constant : Constant  Value=120*pi  VectorParams1D=off  SampleTime=Ts
  Demux : Demux  Outputs=3
  Discrete-Time Integrator : DiscreteIntegrator  SampleTime=Ts  ICPrevOutput=DiscIntNeverNeededParam  ICPrevScaledInput=DiscIntNeverNeededParam
  Gain : Gain  Gain=3
  Gain1 : Gain  Gain=-3
  Inverse Clarke Transform : mcbeeMathTransformLib/Inverse Clarke Transform  PowerInvariant=on  UseWithEmbedded=off  PhaseInput=Two inputs
      settings: LibrarySourceBlock=|
      | ee_sl_lib/Mathematical
      | Transforms/Inverse
      | Clarke Transform
  Inverse Park Transform : eeTransforms/Inverse Park Transform  AxisAlignment=Q-axis  PowerInvariant=off
      settings: LibrarySourceBlock=|
      | ee_sl_lib/Mathematical
      | Transforms/Inverse
      | Park Transform
  Mux : Mux  Inputs=3
  Mux1 : Mux  Inputs=3
  Park Transform : eeTransforms/Park Transform  AxisAlignment=Q-axis  PowerInvariant=off
      settings: LibrarySourceBlock=|
      | ee_sl_lib/Mathematical
      | Transforms/Park Transform
  Product{1..4} (4 alike) : Product
  Product5 : Product  Inputs=/*
  Product6 : Product  Inputs=/*
  Selector : Selector  InputPortWidth=3  IndexOptions=Index vector (dialog)  Indices=1  OutputSizes=1
  Square : Math  Operator=square
  Square1 : Math  Operator=square
  Subsystem : Subsystem
  Sum : Sum
  Sum1 : Sum  Inputs=+-
  Sum2 : Sum
  Terminator6 : Terminator
  Transport Delay2 : TransportDelay  DelayTime=1/180
  Transport Delay3 : TransportDelay  DelayTime=2/180
  I_1ph : Outport
  wires:
  Inverse Clarke Transform/1 -> Selector/1
  Mux1/1 -> Inverse Clarke Transform/1
  Demux/3 -> Terminator6/1
  Clarke Transform/1 -> Demux/1
  Inverse Park Transform/1 -> Clarke Transform/1
  Park Transform/1 -> Subsystem/1(In1)
  Selector/1 -> I_1ph/1
  Mux/1 -> Park Transform/1
  Gain1/1 -> Product3/2, Product1/2
  Gain/1 -> Product2/2, Product4/2
  Transport Delay2/1 -> Mux/2
  meas/1 -> Mux/1, Transport Delay2/1, Transport Delay3/1
  Transport Delay3/1 -> Mux/3
  Subsystem/1(Out1) -> Inverse Park Transform/1
  Discrete-Time Integrator/1 -> Inverse Park Transform/2, Park Transform/2
  Constant/1 -> Discrete-Time Integrator/1
  Product5/1 -> Mux1/1
  Square/1 -> Sum/1
  Product1/1 -> Sum1/1
  Product4/1 -> Sum2/2
  Product6/1 -> Mux1/2
  Demux/1 -> Square/1, Product1/1, Product4/1  "valpha"
  Product2/1 -> Sum1/2
  Sum1/1 -> Product5/2
  "0 "/1 -> Mux1/3
  Q/1 -> Gain/1
  Demux/2 -> Square1/1, Product2/1, Product3/1  "vbeta"
  Product3/1 -> Sum2/1
  Square1/1 -> Sum/2
  P/1 -> Gain1/1
  Sum/1 -> Product6/1, Product5/1
  Sum2/1 -> Product6/2

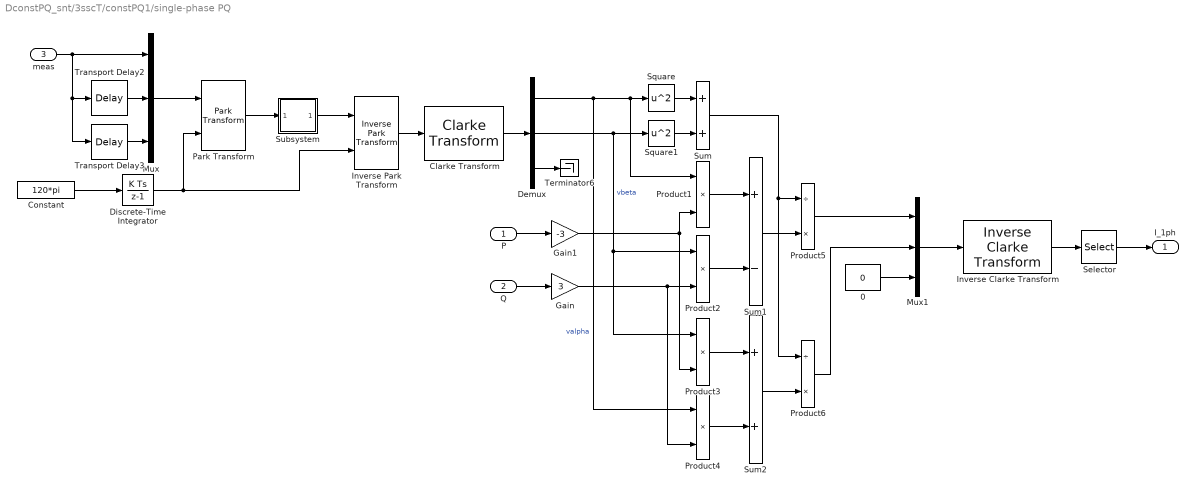
== system DconstPQ_snt/3sscT/constPQ1/single-phase PQ ==
  P : Inport
  Q : Inport  Port=2
  meas : Inport  Port=3
  "0 " : Constant  Value=0  VectorParams1D=off  SampleTime=Ts
  Clarke Transform : mcbeeMathTransformLib/Clarke Transform  PowerInvariant=on  UseWithEmbedded=off  PhaseInput=Two inputs
      settings: LibrarySourceBlock=|
      | ee_sl_lib/Mathematical
      | Transforms/Clarke Transform
  Constant : Constant  Value=120*pi  VectorParams1D=off  SampleTime=Ts
  Demux : Demux  Outputs=3
  Discrete-Time Integrator : DiscreteIntegrator  SampleTime=Ts  ICPrevOutput=DiscIntNeverNeededParam  ICPrevScaledInput=DiscIntNeverNeededParam
  Gain : Gain  Gain=3
  Gain1 : Gain  Gain=-3
  Inverse Clarke Transform : mcbeeMathTransformLib/Inverse Clarke Transform  PowerInvariant=on  UseWithEmbedded=off  PhaseInput=Two inputs
      settings: LibrarySourceBlock=|
      | ee_sl_lib/Mathematical
      | Transforms/Inverse
      | Clarke Transform
  Inverse Park Transform : eeTransforms/Inverse Park Transform  AxisAlignment=Q-axis  PowerInvariant=off
      settings: LibrarySourceBlock=|
      | ee_sl_lib/Mathematical
      | Transforms/Inverse
      | Park Transform
  Mux : Mux  Inputs=3
  Mux1 : Mux  Inputs=3
  Park Transform : eeTransforms/Park Transform  AxisAlignment=Q-axis  PowerInvariant=off
      settings: LibrarySourceBlock=|
      | ee_sl_lib/Mathematical
      | Transforms/Park Transform
  Product{1..4} (4 alike) : Product
  Product5 : Product  Inputs=/*
  Product6 : Product  Inputs=/*
  Selector : Selector  InputPortWidth=3  IndexOptions=Index vector (dialog)  Indices=1  OutputSizes=1
  Square : Math  Operator=square
  Square1 : Math  Operator=square
  Subsystem : Subsystem
  Sum : Sum
  Sum1 : Sum  Inputs=+-
  Sum2 : Sum
  Terminator6 : Terminator
  Transport Delay2 : TransportDelay  DelayTime=1/180
  Transport Delay3 : TransportDelay  DelayTime=2/180
  I_1ph : Outport
  wires:
  Sum2/1 -> Product6/2
  Sum/1 -> Product5/1, Product6/1
  P/1 -> Gain1/1
  Square1/1 -> Sum/2
  Product3/1 -> Sum2/1
  Demux/2 -> Product3/1, Product2/1, Square1/1  "vbeta"
  Q/1 -> Gain/1
  "0 "/1 -> Mux1/3
  Sum1/1 -> Product5/2
  Product2/1 -> Sum1/2
  Demux/1 -> Product4/1, Product1/1, Square/1  "valpha"
  Product6/1 -> Mux1/2
  Product4/1 -> Sum2/2
  Product1/1 -> Sum1/1
  Square/1 -> Sum/1
  Product5/1 -> Mux1/1
  Constant/1 -> Discrete-Time Integrator/1
  Discrete-Time Integrator/1 -> Park Transform/2, Inverse Park Transform/2
  Subsystem/1(Out1) -> Inverse Park Transform/1
  Transport Delay3/1 -> Mux/3
  meas/1 -> Transport Delay3/1, Transport Delay2/1, Mux/1
  Transport Delay2/1 -> Mux/2
  Gain/1 -> Product4/2, Product2/2
  Gain1/1 -> Product1/2, Product3/2
  Mux/1 -> Park Transform/1
  Selector/1 -> I_1ph/1
  Park Transform/1 -> Subsystem/1(In1)
  Inverse Park Transform/1 -> Clarke Transform/1
  Clarke Transform/1 -> Demux/1
  Demux/3 -> Terminator6/1
  Mux1/1 -> Inverse Clarke Transform/1
  Inverse Clarke Transform/1 -> Selector/1

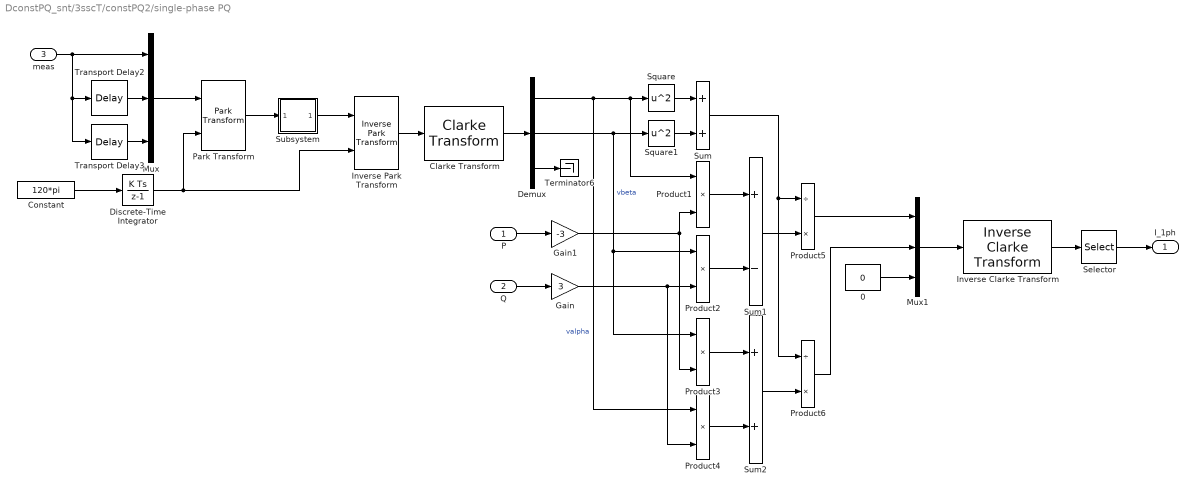
== system DconstPQ_snt/3sscT/constPQ2/single-phase PQ ==
  P : Inport
  Q : Inport  Port=2
  meas : Inport  Port=3
  "0 " : Constant  Value=0  VectorParams1D=off  SampleTime=Ts
  Clarke Transform : mcbeeMathTransformLib/Clarke Transform  PowerInvariant=on  UseWithEmbedded=off  PhaseInput=Two inputs
      settings: LibrarySourceBlock=|
      | ee_sl_lib/Mathematical
      | Transforms/Clarke Transform
  Constant : Constant  Value=120*pi  VectorParams1D=off  SampleTime=Ts
  Demux : Demux  Outputs=3
  Discrete-Time Integrator : DiscreteIntegrator  SampleTime=Ts  ICPrevOutput=DiscIntNeverNeededParam  ICPrevScaledInput=DiscIntNeverNeededParam
  Gain : Gain  Gain=3
  Gain1 : Gain  Gain=-3
  Inverse Clarke Transform : mcbeeMathTransformLib/Inverse Clarke Transform  PowerInvariant=on  UseWithEmbedded=off  PhaseInput=Two inputs
      settings: LibrarySourceBlock=|
      | ee_sl_lib/Mathematical
      | Transforms/Inverse
      | Clarke Transform
  Inverse Park Transform : eeTransforms/Inverse Park Transform  AxisAlignment=Q-axis  PowerInvariant=off
      settings: LibrarySourceBlock=|
      | ee_sl_lib/Mathematical
      | Transforms/Inverse
      | Park Transform
  Mux : Mux  Inputs=3
  Mux1 : Mux  Inputs=3
  Park Transform : eeTransforms/Park Transform  AxisAlignment=Q-axis  PowerInvariant=off
      settings: LibrarySourceBlock=|
      | ee_sl_lib/Mathematical
      | Transforms/Park Transform
  Product{1..4} (4 alike) : Product
  Product5 : Product  Inputs=/*
  Product6 : Product  Inputs=/*
  Selector : Selector  InputPortWidth=3  IndexOptions=Index vector (dialog)  Indices=1  OutputSizes=1
  Square : Math  Operator=square
  Square1 : Math  Operator=square
  Subsystem : Subsystem
  Sum : Sum
  Sum1 : Sum  Inputs=+-
  Sum2 : Sum
  Terminator6 : Terminator
  Transport Delay2 : TransportDelay  DelayTime=1/180
  Transport Delay3 : TransportDelay  DelayTime=2/180
  I_1ph : Outport
  wires:
  Inverse Clarke Transform/1 -> Selector/1
  Mux1/1 -> Inverse Clarke Transform/1
  Demux/3 -> Terminator6/1
  Clarke Transform/1 -> Demux/1
  Inverse Park Transform/1 -> Clarke Transform/1
  Park Transform/1 -> Subsystem/1(In1)
  Selector/1 -> I_1ph/1
  Mux/1 -> Park Transform/1
  Gain1/1 -> Product3/2, Product1/2
  Gain/1 -> Product2/2, Product4/2
  Transport Delay2/1 -> Mux/2
  meas/1 -> Mux/1, Transport Delay2/1, Transport Delay3/1
  Transport Delay3/1 -> Mux/3
  Subsystem/1(Out1) -> Inverse Park Transform/1
  Discrete-Time Integrator/1 -> Inverse Park Transform/2, Park Transform/2
  Constant/1 -> Discrete-Time Integrator/1
  Product5/1 -> Mux1/1
  Square/1 -> Sum/1
  Product1/1 -> Sum1/1
  Product4/1 -> Sum2/2
  Product6/1 -> Mux1/2
  Demux/1 -> Square/1, Product1/1, Product4/1  "valpha"
  Product2/1 -> Sum1/2
  Sum1/1 -> Product5/2
  "0 "/1 -> Mux1/3
  Q/1 -> Gain/1
  Demux/2 -> Square1/1, Product2/1, Product3/1  "vbeta"
  Product3/1 -> Sum2/1
  Square1/1 -> Sum/2
  P/1 -> Gain1/1
  Sum/1 -> Product6/1, Product5/1
  Sum2/1 -> Product6/2

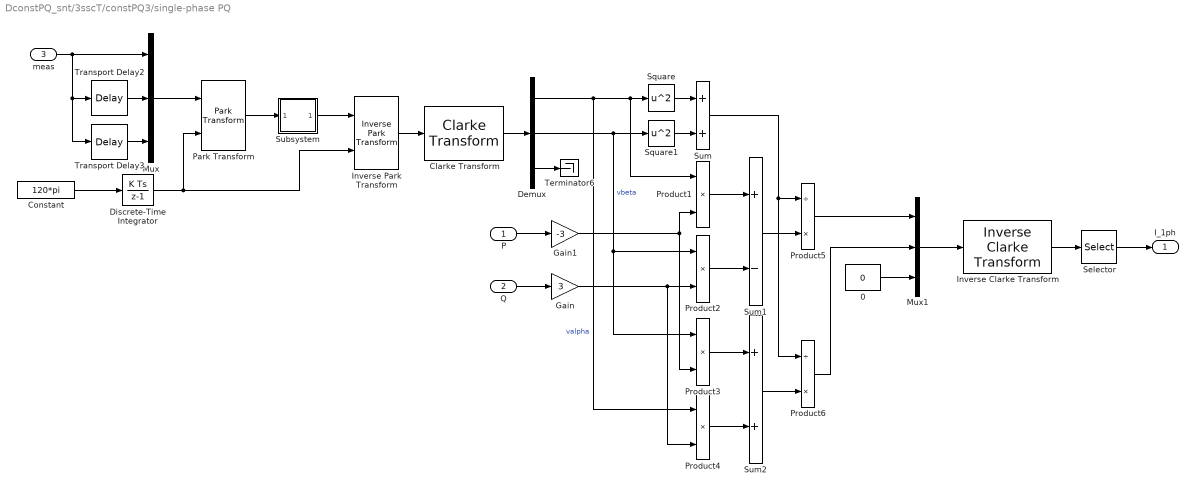
== system DconstPQ_snt/3sscT/constPQ3/single-phase PQ ==
  P : Inport
  Q : Inport  Port=2
  meas : Inport  Port=3
  "0 " : Constant  Value=0  VectorParams1D=off  SampleTime=Ts
  Clarke Transform : mcbeeMathTransformLib/Clarke Transform  PowerInvariant=on  UseWithEmbedded=off  PhaseInput=Two inputs
      settings: LibrarySourceBlock=|
      | ee_sl_lib/Mathematical
      | Transforms/Clarke Transform
  Constant : Constant  Value=120*pi  VectorParams1D=off  SampleTime=Ts
  Demux : Demux  Outputs=3
  Discrete-Time Integrator : DiscreteIntegrator  SampleTime=Ts  ICPrevOutput=DiscIntNeverNeededParam  ICPrevScaledInput=DiscIntNeverNeededParam
  Gain : Gain  Gain=3
  Gain1 : Gain  Gain=-3
  Inverse Clarke Transform : mcbeeMathTransformLib/Inverse Clarke Transform  PowerInvariant=on  UseWithEmbedded=off  PhaseInput=Two inputs
      settings: LibrarySourceBlock=|
      | ee_sl_lib/Mathematical
      | Transforms/Inverse
      | Clarke Transform
  Inverse Park Transform : eeTransforms/Inverse Park Transform  AxisAlignment=Q-axis  PowerInvariant=off
      settings: LibrarySourceBlock=|
      | ee_sl_lib/Mathematical
      | Transforms/Inverse
      | Park Transform
  Mux : Mux  Inputs=3
  Mux1 : Mux  Inputs=3
  Park Transform : eeTransforms/Park Transform  AxisAlignment=Q-axis  PowerInvariant=off
      settings: LibrarySourceBlock=|
      | ee_sl_lib/Mathematical
      | Transforms/Park Transform
  Product{1..4} (4 alike) : Product
  Product5 : Product  Inputs=/*
  Product6 : Product  Inputs=/*
  Selector : Selector  InputPortWidth=3  IndexOptions=Index vector (dialog)  Indices=1  OutputSizes=1
  Square : Math  Operator=square
  Square1 : Math  Operator=square
  Subsystem : Subsystem
  Sum : Sum
  Sum1 : Sum  Inputs=+-
  Sum2 : Sum
  Terminator6 : Terminator
  Transport Delay2 : TransportDelay  DelayTime=1/180
  Transport Delay3 : TransportDelay  DelayTime=2/180
  I_1ph : Outport
  wires:
  Sum2/1 -> Product6/2
  Sum/1 -> Product5/1, Product6/1
  P/1 -> Gain1/1
  Square1/1 -> Sum/2
  Product3/1 -> Sum2/1
  Demux/2 -> Product3/1, Product2/1, Square1/1  "vbeta"
  Q/1 -> Gain/1
  "0 "/1 -> Mux1/3
  Sum1/1 -> Product5/2
  Product2/1 -> Sum1/2
  Demux/1 -> Product4/1, Product1/1, Square/1  "valpha"
  Product6/1 -> Mux1/2
  Product4/1 -> Sum2/2
  Product1/1 -> Sum1/1
  Square/1 -> Sum/1
  Product5/1 -> Mux1/1
  Constant/1 -> Discrete-Time Integrator/1
  Discrete-Time Integrator/1 -> Park Transform/2, Inverse Park Transform/2
  Subsystem/1(Out1) -> Inverse Park Transform/1
  Transport Delay3/1 -> Mux/3
  meas/1 -> Transport Delay3/1, Transport Delay2/1, Mux/1
  Transport Delay2/1 -> Mux/2
  Gain/1 -> Product4/2, Product2/2
  Gain1/1 -> Product1/2, Product3/2
  Mux/1 -> Park Transform/1
  Selector/1 -> I_1ph/1
  Park Transform/1 -> Subsystem/1(In1)
  Inverse Park Transform/1 -> Clarke Transform/1
  Clarke Transform/1 -> Demux/1
  Demux/3 -> Terminator6/1
  Mux1/1 -> Inverse Clarke Transform/1
  Inverse Clarke Transform/1 -> Selector/1

== system DconstPQ_snt/1sscT/constPQ1/single-phase PQ/Subsystem ==
  In1 : Inport
  Discrete-Time Integrator : DiscreteIntegrator  gainval=1/Ts/20  InitialCondition=2000  SampleTime=-1  ICPrevOutput=DiscIntNeverNeededParam  ICPrevScaledInput=DiscIntNeverNeededParam
  Sum : Sum  Inputs=|+-
  Out1 : Outport
  wires:
  In1/1 -> Sum/1
  Sum/1 -> Discrete-Time Integrator/1
  Discrete-Time Integrator/1 -> Sum/2, Out1/1

== system DconstPQ_snt/2sscT/constPQ/single-phase PQ/Subsystem ==
  In1 : Inport
  Discrete-Time Integrator : DiscreteIntegrator  gainval=1/Ts/20  InitialCondition=2000  SampleTime=-1  ICPrevOutput=DiscIntNeverNeededParam  ICPrevScaledInput=DiscIntNeverNeededParam
  Sum : Sum  Inputs=|+-
  Out1 : Outport
  wires:
  In1/1 -> Sum/1
  Sum/1 -> Discrete-Time Integrator/1
  Discrete-Time Integrator/1 -> Sum/2, Out1/1

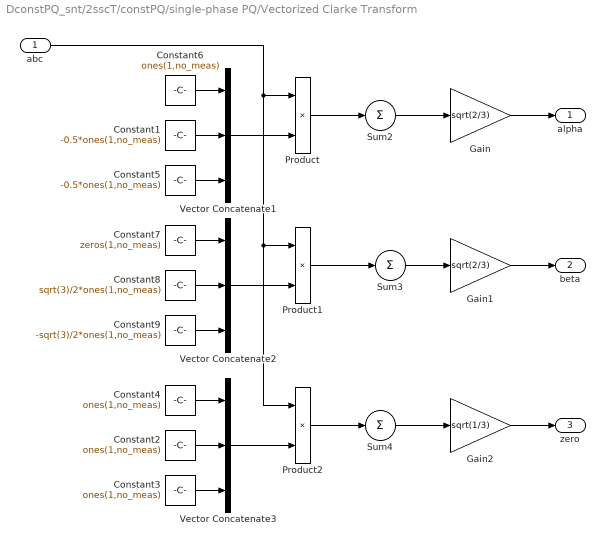
== system DconstPQ_snt/2sscT/constPQ/single-phase PQ/Vectorized Clarke Transform ==
  abc : Inport
  Constant1 : Constant  Value=-0.5*ones(1,no_meas)  VectorParams1D=off  SampleTime=Ts
  Constant{2..4,6} (4 alike) : Constant  Value=ones(1,no_meas)  VectorParams1D=off  SampleTime=Ts
  Constant5 : Constant  Value=-0.5*ones(1,no_meas)  VectorParams1D=off  SampleTime=Ts
  Constant7 : Constant  Value=zeros(1,no_meas)  VectorParams1D=off  SampleTime=Ts
  Constant8 : Constant  Value=sqrt(3)/2*ones(1,no_meas)  VectorParams1D=off  SampleTime=Ts
  Constant9 : Constant  Value=-sqrt(3)/2*ones(1,no_meas)  VectorParams1D=off  SampleTime=Ts
  Gain : Gain  Gain=sqrt(2/3)
  Gain1 : Gain  Gain=sqrt(2/3)
  Gain2 : Gain  Gain=sqrt(1/3)
  Product : Product
  Product1 : Product
  Product2 : Product
  Sum2 : Sum  Inputs=1  CollapseMode=Specified dimension  InputSameDT=on  SaturateOnIntegerOverflow=on  OutDataTypeStr=Inherit: Same as first input
  Sum3 : Sum  Inputs=1  CollapseMode=Specified dimension  InputSameDT=on  SaturateOnIntegerOverflow=on  OutDataTypeStr=Inherit: Same as first input
  Sum4 : Sum  Inputs=1  CollapseMode=Specified dimension  InputSameDT=on  SaturateOnIntegerOverflow=on  OutDataTypeStr=Inherit: Same as first input
  Vector Concatenate1 : Concatenate  NumInputs=3  Mode=Multidimensional array
  Vector Concatenate2 : Concatenate  NumInputs=3  Mode=Multidimensional array
  Vector Concatenate3 : Concatenate  NumInputs=3  Mode=Multidimensional array
  alpha : Outport  VectorParamsAs1DForOutWhenUnconnected=off
  beta : Outport  Port=2  VectorParamsAs1DForOutWhenUnconnected=off
  zero : Outport  Port=3  VectorParamsAs1DForOutWhenUnconnected=off
  wires:
  Gain/1 -> alpha/1
  Gain1/1 -> beta/1
  Gain2/1 -> zero/1
  Sum2/1 -> Gain/1
  Sum4/1 -> Gain2/1
  Sum3/1 -> Gain1/1
  Product2/1 -> Sum4/1
  Product1/1 -> Sum3/1
  Product/1 -> Sum2/1
  Vector Concatenate1/1 -> Product/2
  Vector Concatenate2/1 -> Product1/2
  Vector Concatenate3/1 -> Product2/2
  Constant3/1 -> Vector Concatenate3/3
  Constant2/1 -> Vector Concatenate3/2
  Constant4/1 -> Vector Concatenate3/1
  abc/1 -> Product/1, Product1/1, Product2/1
  Constant6/1 -> Vector Concatenate1/1
  Constant1/1 -> Vector Concatenate1/2
  Constant5/1 -> Vector Concatenate1/3
  Constant7/1 -> Vector Concatenate2/1
  Constant8/1 -> Vector Concatenate2/2
  Constant9/1 -> Vector Concatenate2/3

== system DconstPQ_snt/2sscT/constPQ/single-phase PQ/Vectorized PQ meas ==
  V : Inport
  I : Inport  Port=2
  Product1 : Product  InputSameDT=on  SaturateOnIntegerOverflow=on  OutDataTypeStr=Inherit: Same as first input
  Product3 : Product  InputSameDT=on  SaturateOnIntegerOverflow=on  OutDataTypeStr=Inherit: Same as first input
  Sum1 : Sum  Inputs=1  CollapseMode=Specified dimension  InputSameDT=on  SaturateOnIntegerOverflow=on  OutDataTypeStr=Inherit: Same as first input
  Sum2 : Sum  Inputs=1  CollapseMode=Specified dimension  InputSameDT=on  SaturateOnIntegerOverflow=on  OutDataTypeStr=Inherit: Same as first input
  Sum4 : Sum  Inputs=+-  InputSameDT=on  SaturateOnIntegerOverflow=on  OutDataTypeStr=Inherit: Same as first input
  pu->V : Gain  Gain=1/sqrt(3)  SaturateOnIntegerOverflow=on  OutDataTypeStr=Inherit: Same as input  ParamDataTypeStr=Inherit: Same as input
  pu->V1 : Gain  Gain=[0 1 0;0 0 1;1 0 0]  Multiplication=Matrix(K*u)  SaturateOnIntegerOverflow=on  OutDataTypeStr=Inherit: Same as input  ParamDataTypeStr=Inherit: Same as input
  pu->V2 : Gain  Gain=[0 1 0;0 0 1;1 0 0]  Multiplication=Matrix(K*u)  SaturateOnIntegerOverflow=on  OutDataTypeStr=Inherit: Same as input  ParamDataTypeStr=Inherit: Same as input
  P : Outport  VectorParamsAs1DForOutWhenUnconnected=off
  Q : Outport  Port=2  VectorParamsAs1DForOutWhenUnconnected=off
  wires:
  pu->V/1 -> Q/1
  Sum1/1 -> pu->V/1
  Product3/1 -> Sum1/1
  Product1/1 -> Sum2/1
  V/1 -> Sum4/1, pu->V1/1, Product1/1  "VV1"
  I/1 -> Product3/2, Product1/2
  Sum2/1 -> P/1
  pu->V1/1 -> Sum4/2
  Sum4/1 -> pu->V2/1  "VV2"
  pu->V2/1 -> Product3/1

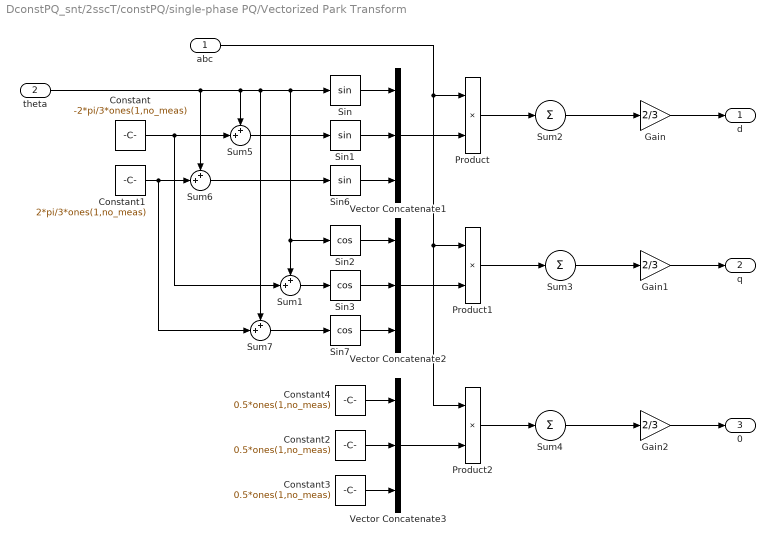
== system DconstPQ_snt/2sscT/constPQ/single-phase PQ/Vectorized Park Transform ==
  abc : Inport
  theta : Inport  Port=2
  Constant : Constant  Value=-2*pi/3*ones(1,no_meas)  VectorParams1D=off  SampleTime=Ts
  Constant1 : Constant  Value=2*pi/3*ones(1,no_meas)  VectorParams1D=off  SampleTime=Ts
  Constant2 : Constant  Value=0.5*ones(1,no_meas)  VectorParams1D=off  SampleTime=Ts
  Constant3 : Constant  Value=0.5*ones(1,no_meas)  VectorParams1D=off  SampleTime=Ts
  Constant4 : Constant  Value=0.5*ones(1,no_meas)  VectorParams1D=off  SampleTime=Ts
  Gain : Gain  Gain=2/3
  Gain1 : Gain  Gain=2/3
  Gain2 : Gain  Gain=2/3
  Product : Product
  Product1 : Product
  Product2 : Product
  Sin : Trigonometry
  Sin1 : Trigonometry
  Sin2 : Trigonometry  Operator=cos
  Sin3 : Trigonometry  Operator=cos
  Sin6 : Trigonometry
  Sin7 : Trigonometry  Operator=cos
  Sum{1,5..7} (4 alike) : Sum  Inputs=++|
  Sum2 : Sum  Inputs=1  CollapseMode=Specified dimension  InputSameDT=on  SaturateOnIntegerOverflow=on  OutDataTypeStr=Inherit: Same as first input
  Sum3 : Sum  Inputs=1  CollapseMode=Specified dimension  InputSameDT=on  SaturateOnIntegerOverflow=on  OutDataTypeStr=Inherit: Same as first input
  Sum4 : Sum  Inputs=1  CollapseMode=Specified dimension  InputSameDT=on  SaturateOnIntegerOverflow=on  OutDataTypeStr=Inherit: Same as first input
  Vector Concatenate1 : Concatenate  NumInputs=3  Mode=Multidimensional array
  Vector Concatenate2 : Concatenate  NumInputs=3  Mode=Multidimensional array
  Vector Concatenate3 : Concatenate  NumInputs=3  Mode=Multidimensional array
  d : Outport  VectorParamsAs1DForOutWhenUnconnected=off
  q : Outport  Port=2  VectorParamsAs1DForOutWhenUnconnected=off
  0 : Outport  Port=3  VectorParamsAs1DForOutWhenUnconnected=off
  wires:
  Gain/1 -> d/1
  Gain1/1 -> q/1
  Gain2/1 -> 0/1
  Sum2/1 -> Gain/1
  Sum4/1 -> Gain2/1
  Sum3/1 -> Gain1/1
  Product2/1 -> Sum4/1
  Product1/1 -> Sum3/1
  Product/1 -> Sum2/1
  Vector Concatenate1/1 -> Product/2
  Vector Concatenate2/1 -> Product1/2
  Vector Concatenate3/1 -> Product2/2
  Constant3/1 -> Vector Concatenate3/3
  Sin7/1 -> Vector Concatenate2/3
  Sin6/1 -> Vector Concatenate1/3
  Constant2/1 -> Vector Concatenate3/2
  Constant4/1 -> Vector Concatenate3/1
  Sin2/1 -> Vector Concatenate2/1
  Sin3/1 -> Vector Concatenate2/2
  Sin1/1 -> Vector Concatenate1/2
  Sin/1 -> Vector Concatenate1/1
  abc/1 -> Product/1, Product1/1, Product2/1
  Sum5/1 -> Sin1/1
  Sum6/1 -> Sin6/1
  Constant/1 -> Sum1/2, Sum5/2
  Constant1/1 -> Sum7/2, Sum6/2
  Sum1/1 -> Sin3/1
  Sum7/1 -> Sin7/1
  theta/1 -> Sum6/1, Sum5/1, Sin2/1, Sum1/1, Sin/1, Sum7/1
